simulink model "cruiseSym"  (Simulink 10.0)
settings: Solver=VariableStepAuto  StartTime=0.0  StopTime=100  RelTol=1e-3
undefined symbols (not defined in the file): A, a3, Be, Cd, Cr, g, i, m, P, sgn, the, Tm, wm
libraries: simulink_extras x1
settings Model: Creator=aravind  LastModifiedBy=aravind
settings DataIOCC: SaveFormat=Dataset  ReturnWorkspaceOutputs=on
settings OptimizationCC: LifeSpan=auto
settings DebuggingCC: UnderspecifiedInitializationDetection=Simplified  MergeDetectMultiDrivingBlocksExec=error  SFUnexpectedBacktrackingDiag=error  SFNoUnconditionalDefaultTransitionDiag=error  SFExecutionAtInitializationDiag=warning  ArithmeticOperatorsInVariantConditions=error
settings HardwareCC: ProdBitPerPointer=64  ProdBitPerSizeT=64  ProdBitPerPtrDiffT=64  ProdLargestAtomicFloat=Float  ProdIntDivRoundTo=Zero  ProdEndianess=LittleEndian  ProdWordSize=64  ProdHWDeviceType=Intel->x86-64 (Windows64)
settings ModelReferenceCC: PropagateSignalLabelsOutOfModel=on
settings SFSimCC: SimUseLocalCustomCode=on  CustomCodeUndefinedFunction=FilterOut
settings RTWCC: RTWUseLocalCustomCode=on
settings CodeAppCC: StateflowObjectComments=off
settings GRTTargetCC: TargetLangStandard=C99 (ISO)  CombineOutputUpdateFcns=on  GRTInterface=off
settings ConfigComp: CovMetricSettings=dwe  CovHtmlReporting=off  CovSaveCumulativeToWorkspaceVar=off  CovSaveSingleToWorkspaceVar=off

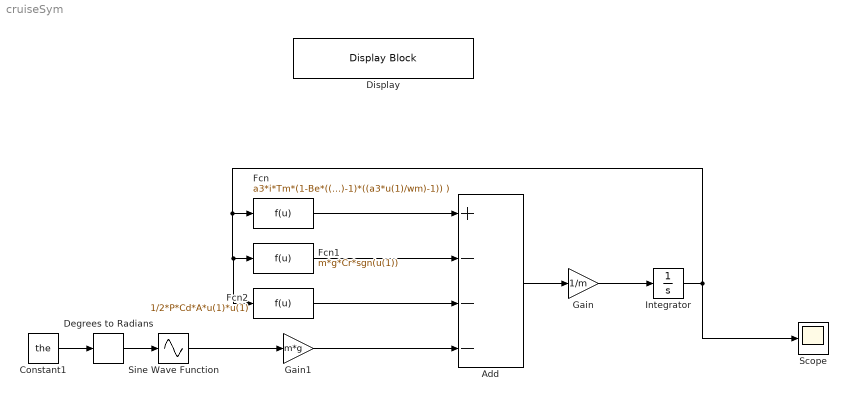
== system cruiseSym ==
  Add : Sum  Inputs=+---
  Constant1 : Constant  Value=the
  Degrees to Radians : simulink_extras/Transformations/Degrees to Radians
  Display : DisplayBlock  LabelPosition=Hide  Format=short  Transparency=1
  Fcn : Fcn  Expr=a3*i*Tm*(1-Be*(((a3*u(1)/wm)-1)*((a3*u(1)/wm)-1)) )
  Fcn1 : Fcn  Expr=m*g*Cr*sgn(u(1))
  Fcn2 : Fcn  Expr=1/2*P*Cd*A*u(1)*u(1)
  Gain : Gain  Gain=1/m
  Gain1 : Gain  Gain=m*g
  Integrator : Integrator
  Scope : Scope
  Sine Wave Function : Sin  TimeSource=Use external signal  SampleTime=0
  wires:
  Fcn/1 -> Add/1
  Fcn1/1 -> Add/2
  Fcn2/1 -> Add/3
  Gain1/1 -> Add/4
  Add/1 -> Gain/1
  Sine Wave Function/1 -> Gain1/1
  Gain/1 -> Integrator/1
  Integrator/1 -> Fcn2/1, Fcn1/1, Fcn/1, Scope/1
  Degrees to Radians/1 -> Sine Wave Function/1
  Constant1/1 -> Degrees to Radians/1
